simulink model "untitled1"  (R2024b)
settings: Solver=VariableStepAuto  StartTime=0.0  StopTime=10.0  RelTol=1e-3
libraries: spsSeriesRLCLoadLib x12, spsUniversalBridgeLib x6, spsAsynchronousMachineSIUnitsLib x4, spsCurrentMeasurementLib x4, spsIdealSwitchLib x4, spsThreePhaseVIMeasurementLib x2, spsControlledVoltageSourceLib x1, spsMultiWindingTransformerLib x1, spsThreePhaseTransformerInductanceMatrixTypeTwoWindingsLib x1, spsVoltageMeasurementLib x1
settings Model: Creator=HFUT2  LastModifiedBy=HFUT2

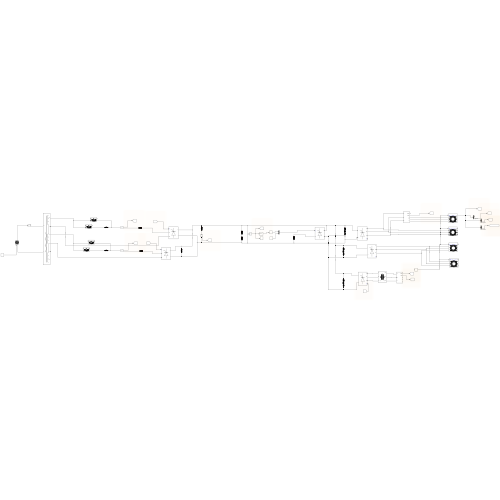
[thumbnail: Simulink's stored preview of the top-level diagram]
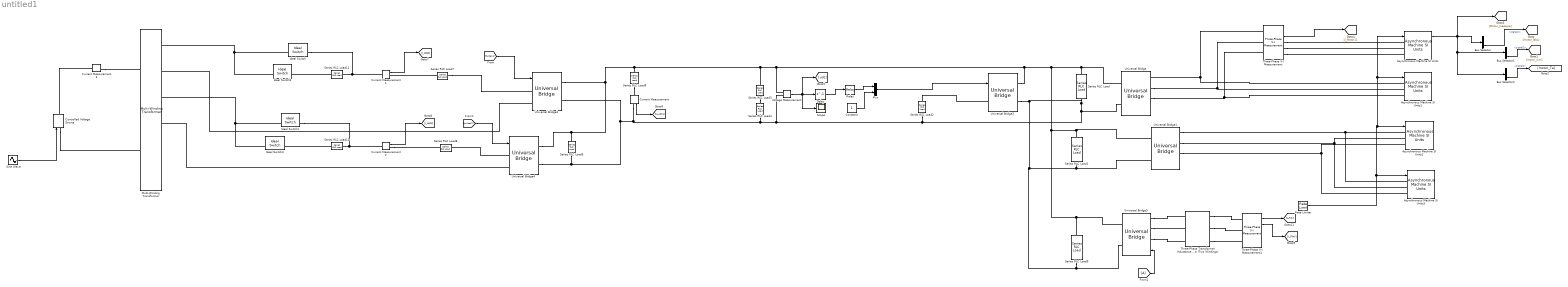
== system untitled1 ==
  Asynchronous Machine SI Units{,1..3} (4 alike) : spsAsynchronousMachineSIUnitsLib/Asynchronous Machine SI Units  RotorType=Wound  PresetModel=No  MechanicalLoad=Torque Tm  ShowDetailedParameters=on  ReferenceFrame=Rotor  Units=SI  MeasurementBus=off  NominalParameters=[1.845e+04 400 50]  VoltageRatio=1  Stator=[0.5968 0.0003495]  Rotor=[0.6258 0.005473]  Cage1=[0.4155 0.002066]  Cage2=[0.4168 0.0003495]  Lm=0.0354  Mechanical=[0.05 0.005879 2]  PolePairs=2  InitialConditions=[0 0 0 0 0 0 0 0]  SimulateSaturation=off  Saturation=[14.03593122, 27.81365428, 53.79336849, 72.68890987, 97.98006896, 148.6815601, 215.7428561, 302.9841135, 428.7778367 ; 230, 322, 414, 460, 506, 552, 598, 644, 690]  LoadFlowParameters=1492000  TsPowergui=0  TsBlock=-1  IterativeModel=Trapezoidal non iterative  IterativeDiscreteModel=Trapezoidal non iterative  Pmec=1.492e+006
  Bus Selector : BusSelector  OutputSignals=signal1,signal2
  Bus Selector1 : BusSelector  OutputSignals=signal1,signal2
  Bus Selector2 : BusSelector  OutputSignals=signal1,signal2
  Constant : Constant
  Controlled Voltage Source : spsControlledVoltageSourceLib/Controlled Voltage Source  Initialize=on  Source_Type=AC  Amplitude=0  Phase=0  Frequency=0  Measurements=None
  Current Measurement{,1..3} (4 alike) : spsCurrentMeasurementLib/Current Measurement  PhasorSimulation=off  OutputType=Complex  PSBequivalent=0
  Delay : Delay  DelayLength=1  InitialCondition=0
  From2 : From
  Ideal Switch{,1..3} (4 alike) : spsIdealSwitchLib/Ideal Switch  Ron=0.001  Lon=0  IC=0  Rs=1e5  Cs=inf  Measurements=on
  Multi-Winding Transformer : spsMultiWindingTransformerLib/Multi-Winding Transformer  LeftWindings=1  RightWindings=3  TappedWindings=no taps  NumberOfTaps=2  SetSaturation=off  Hysteresis=off  DataFile='hysteresis.mat'  Measurements=None  UNITS=pu  NominalPower=[75e3 60]  NominalVoltages="[ 14400  120  120 120 ]"  WindingResistances="[ 0.005  0.005  0.005  0.005]"  WindingInductances="[ 0.02  0.02  0.02  0.02 ]"  Rm=50  Lm=50  Saturation=[ 0,0 ; 0.0024,1.2 ; 1.0,1.52 ]  SpecifyInitialFlux=off  InitialFlux=0  BreakLoop=off  DiscreteSolver=Trapezoidal iterative  DataType=off  TransfoNumber=1
      settings: LibrarySourceBlock=|
      | sps_lib/Power Grid Elements/Multi-Winding
      | Transformer
  Mux : Mux  Inputs=2
  Rate Limiter : RateLimiter  SampleTimeMode=inherited
  Relay : Relay
  Scope : Scope
  Series RLC Load{,1..9,11..12} (12 alike) : spsSeriesRLCLoadLib/Series RLC Load  LConnTagsString=a  RConnTagsString=__new0  NominalVoltage=1000  NominalFrequency=60  ActivePower=10e3  InductivePower=100  CapacitivePower=100  Setx0=off  InitialVoltage=0  SetiL0=off  InitialCurrent=0  Measurements=None  LoadType=constant Z
  Sine Wave : Sin  SampleTime=0
  Three-Phase V-I Measurement : spsThreePhaseVIMeasurementLib/Three-Phase V-I Measurement  VoltageMeasurement=phase-to-ground  SetLabelV=off  LabelV=Vabc  Vpu=off  VpuLL=off  CurrentMeasurement=yes  SetLabelI=off  LabelI=Iabc  Ipu=off  Pbase=100e6  Vbase=500e3  OutputType=Complex  PhasorSimulation=off  PSBequivalent=0
  Three-Phase V-I Measurement1 : spsThreePhaseVIMeasurementLib/Three-Phase V-I Measurement  VoltageMeasurement=phase-to-ground  SetLabelV=off  LabelV=Vabc  Vpu=off  VpuLL=off  CurrentMeasurement=yes  SetLabelI=off  LabelI=Iabc  Ipu=off  Pbase=100e6  Vbase=500e3  OutputType=Complex  PhasorSimulation=off  PSBequivalent=0
  Three-Phase Transformer Inductance Matrix Type (Two Windings) : spsThreePhaseTransformerInductanceMatrixTypeTwoWindingsLib/Three-Phase Transformer Inductance Matrix Type (Two Windings)  CoreType=Three-limb or five-limb core  Winding1Connection=Yg  Winding2Connection=Yg  AutoTransformer=off  Measurements=None  NominalPower=[100e3, 60]  VLLnom=[2400, 600]  WindingResistances=[0.01, 0.01]  NoLoadIexcPos=2  NoLoadPlossPos=1000  ShortCircuitReactancePos=0.06  ShortCircuitReactancePosAuto=0.06  NoLoadIexcZero=100  NoLoadPlossZero=1500  ShortCircuitReactanceZero=0.03  ShortCircuitReactanceZeroAuto=0.03
      settings: LibrarySourceBlock=|
      | sps_lib/Power Grid Elements/Three-Phase Transformer
      | Inductance Matrix Type
      | (Two Windings)
  Universal Bridge : spsUniversalBridgeLib/Universal Bridge  Arms=3  SnubberResistance=1e5  SnubberCapacitance=inf  Device=Thyristors  Ron=1e-3  Lon=0  ForwardVoltages="[  0  0  ]"  ForwardVoltage=0  GTOparameters=[ 10e-6 , 20e-6 ]  IGBTparameters=[ 1e-6 , 2e-6 ]  Measurements=None  Measurements_2=None  converterType=Rectifier
  Universal Bridge1 : spsUniversalBridgeLib/Universal Bridge  Arms=3  SnubberResistance=1e5  SnubberCapacitance=inf  Device=Thyristors  Ron=1e-3  Lon=0  ForwardVoltages="[  0  0  ]"  ForwardVoltage=0  GTOparameters=[ 10e-6 , 20e-6 ]  IGBTparameters=[ 1e-6 , 2e-6 ]  Measurements=None  Measurements_2=None  converterType=Rectifier
  Universal Bridge2 : spsUniversalBridgeLib/Universal Bridge  Arms=1  SnubberResistance=1e5  SnubberCapacitance=inf  Device=Thyristors  Ron=1e-3  Lon=0  ForwardVoltages="[  0  0  ]"  ForwardVoltage=0  GTOparameters=[ 10e-6 , 20e-6 ]  IGBTparameters=[ 1e-6 , 2e-6 ]  Measurements=None  Measurements_2=None  converterType=Rectifier
  Universal Bridge3 : spsUniversalBridgeLib/Universal Bridge  Arms=2  SnubberResistance=1e5  SnubberCapacitance=inf  Device=Thyristors  Ron=1e-3  Lon=0  ForwardVoltages="[  0  0  ]"  ForwardVoltage=0  GTOparameters=[ 10e-6 , 20e-6 ]  IGBTparameters=[ 1e-6 , 2e-6 ]  Measurements=None  Measurements_2=None  converterType=Rectifier
  Universal Bridge4 : spsUniversalBridgeLib/Universal Bridge  Arms=2  SnubberResistance=1e5  SnubberCapacitance=inf  Device=Thyristors  Ron=1e-3  Lon=0  ForwardVoltages="[  0  0  ]"  ForwardVoltage=0  GTOparameters=[ 10e-6 , 20e-6 ]  IGBTparameters=[ 1e-6 , 2e-6 ]  Measurements=None  Measurements_2=None  converterType=Rectifier
  Universal Bridge5 : spsUniversalBridgeLib/Universal Bridge  Arms=3  SnubberResistance=1e5  SnubberCapacitance=inf  Device=Thyristors  Ron=1e-3  Lon=0  ForwardVoltages="[  0  0  ]"  ForwardVoltage=0  GTOparameters=[ 10e-6 , 20e-6 ]  IGBTparameters=[ 1e-6 , 2e-6 ]  Measurements=None  Measurements_2=None  converterType=Rectifier
  Voltage Measurement : spsVoltageMeasurementLib/Voltage Measurement  PhasorSimulation=off  OutputType=Complex  PSBequivalent=0
  wires:
  Asynchronous Machine SI Units/1 -> Bus Selector2/1, Bus Selector1/1, Bus Selector/1, [Motor_measure]
  Bus Selector/2 -> [motor_labc]  "<signal2>"
  Bus Selector1/2 -> [motor_wm]  "<signal2>"
  Bus Selector2/2 -> [motor_Te]  "<signal2>"
  Three-Phase V-I Measurement/2 -> [I_Motor1]
  Rate Limiter/1 -> Asynchronous Machine SI Units1/1, Asynchronous Machine SI Units/1, Asynchronous Machine SI Units2/1, Asynchronous Machine SI Units3/1
  Delay/1 -> Relay/1
  Relay/1 -> Mux/1
  Constant/1 -> Mux/2
  Mux/1 -> Universal Bridge2/1
  Voltage Measurement/1 -> Scope/1, Delay/1, [udc]
  Current Measurement/1 -> [ic_4QS1]
  [Pulse11] -> Universal Bridge3/1
  [pulse12] -> Universal Bridge4/1
  Current Measurement1/1 -> [i_4qs1]
  Current Measurement2/1 -> [i_4qs2]
  Sine Wave/1 -> Controlled Voltage Source/1
  From2/1 -> Universal Bridge5/1
  Three-Phase V-I Measurement1/1 -> [U_FINV]
  Three-Phase V-I Measurement1/2 -> [I_FINV]
  connections:
  Three-Phase V-I Measurement/RConn1 -- Asynchronous Machine SI Units/LConn1
  Three-Phase V-I Measurement/RConn2 -- Asynchronous Machine SI Units/LConn2
  Three-Phase V-I Measurement/RConn3 -- Asynchronous Machine SI Units/LConn3
  Universal Bridge1/LConn3 -- Asynchronous Machine SI Units3/LConn1 -- Asynchronous Machine SI Units2/LConn1
  Universal Bridge1/LConn2 -- Asynchronous Machine SI Units2/LConn2 -- Asynchronous Machine SI Units3/LConn2
  Universal Bridge1/LConn1 -- Asynchronous Machine SI Units2/LConn3 -- Asynchronous Machine SI Units3/LConn3
  Asynchronous Machine SI Units1/LConn1 -- Three-Phase V-I Measurement/LConn1 -- Universal Bridge/LConn3
  Universal Bridge/LConn1 -- Three-Phase V-I Measurement/LConn3 -- Asynchronous Machine SI Units1/LConn3
  Three-Phase V-I Measurement/LConn2 -- Asynchronous Machine SI Units1/LConn2 -- Universal Bridge/LConn2
  Universal Bridge1/RConn2 -- Universal Bridge5/RConn2 -- Series RLC Load9/LConn1 -- Series RLC Load6/LConn1 -- Universal Bridge4/RConn1 -- Universal Bridge3/RConn1 -- Series RLC Load5/LConn1 -- Series RLC Load3/LConn1 -- Voltage Measurement/LConn1 -- Universal Bridge2/RConn1 -- Series RLC Load/LConn1 -- Universal Bridge/RConn2 -- Series RLC Load1/LConn1
  Universal Bridge1/RConn1 -- Series RLC Load9/RConn1 -- Universal Bridge5/RConn1 -- Series RLC Load6/RConn1 -- Universal Bridge4/RConn2 -- Universal Bridge3/RConn2 -- Current Measurement/RConn1 -- Series RLC Load4/RConn1 -- Voltage Measurement/LConn2 -- Series RLC Load2/RConn1 -- Universal Bridge/RConn1 -- Series RLC Load/RConn1 -- Universal Bridge2/RConn2 -- Series RLC Load1/RConn1
  Universal Bridge2/LConn1 -- Series RLC Load2/LConn1
  Series RLC Load3/RConn1 -- Series RLC Load4/LConn1
  Series RLC Load5/RConn1 -- Current Measurement/LConn1
  Series RLC Load7/LConn1 -- Universal Bridge3/LConn1
  Universal Bridge4/LConn1 -- Series RLC Load8/LConn1
  Current Measurement2/RConn1 -- Series RLC Load8/RConn1
  Series RLC Load7/RConn1 -- Current Measurement1/RConn1
  Current Measurement1/LConn1 -- Ideal Switch/RConn1 -- Series RLC Load11/LConn1
  Current Measurement2/LConn1 -- Ideal Switch1/RConn1 -- Series RLC Load12/LConn1
  Series RLC Load11/RConn1 -- Ideal Switch2/RConn1
  Series RLC Load12/RConn1 -- Ideal Switch3/RConn1
  Ideal Switch/LConn1 -- Ideal Switch2/LConn1 -- Multi-Winding Transformer/RConn1
  Universal Bridge3/LConn2 -- Multi-Winding Transformer/RConn2
  Ideal Switch1/LConn1 -- Ideal Switch3/LConn1 -- Multi-Winding Transformer/RConn3
  Universal Bridge4/LConn2 -- Multi-Winding Transformer/RConn4
  Current Measurement3/RConn1 -- Multi-Winding Transformer/LConn1
  Controlled Voltage Source/RConn1 -- Current Measurement3/LConn1
  Controlled Voltage Source/LConn1 -- Multi-Winding Transformer/LConn2
  Universal Bridge5/LConn3 -- Three-Phase Transformer Inductance Matrix Type (Two Windings)/LConn1
  Universal Bridge5/LConn2 -- Three-Phase Transformer Inductance Matrix Type (Two Windings)/LConn2
  Universal Bridge5/LConn1 -- Three-Phase Transformer Inductance Matrix Type (Two Windings)/LConn3
  Three-Phase Transformer Inductance Matrix Type (Two Windings)/RConn1 -- Three-Phase V-I Measurement1/LConn1
  Three-Phase Transformer Inductance Matrix Type (Two Windings)/RConn2 -- Three-Phase V-I Measurement1/LConn2
  Three-Phase Transformer Inductance Matrix Type (Two Windings)/RConn3 -- Three-Phase V-I Measurement1/LConn3
